simulink model "buck_hvoltage_discrete"  (R2014a)
settings: Solver=ode45  StartTime=0.0  StopTime=5*Tmax  RelTol=1e-3
values from neighbouring files (symbols this model uses):
  a00c = sys(1).Ac(1,1)    [parameters.m]
  a00d = sys(1).Ad(1,1)    [parameters.m]
  a00o = sys(1).Ao(1,1)    [parameters.m]
  a01c = sys(1).Ac(1,2)    [parameters.m]
  a01d = sys(1).Ad(1,2)    [parameters.m]
  a01o = sys(1).Ao(1,2)    [parameters.m]
  a10c = sys(1).Ac(2,1)    [parameters.m]
  a10d = sys(1).Ad(2,1)    [parameters.m]
  a10o = sys(1).Ao(2,1)    [parameters.m]
  a11c = sys(1).Ac(2,2)    [parameters.m]
  a11d = sys(1).Ad(2,2)    [parameters.m]
  a11o = sys(1).Ao(2,2)    [parameters.m]
  b0c = sys(1).Bc(1)    [parameters.m]
  b0d = sys(1).Bd(1)    [parameters.m]
  b0o = sys(1).Bo(1)    [parameters.m]
  b1c = sys(1).Bc(2)    [parameters.m]
  b1d = sys(1).Bd(2)    [parameters.m]
  b1o = sys(1).Bo(2)    [parameters.m]
  D = cr*Vref/(cr*Vref + Vs)    (= 0.489795918367)    [parameters.m]
  i0 = 4.5    [parameters.m]
  T = 4e-6    (= 4e-06)    [parameters.m]
  v0 = 48    [parameters.m]
  Vref = 15    [parameters.m]    (also in parameters_dcmicrogrid.m = [48 48]; parameters_dcmicrogrid_hynger.m = [48 48])
  Vtol = Vref / 200    (= 0.075)    [parameters.m]
libraries: simulink x1
settings Model: BufferReuse=off  Creator=Luan Nguyen  LastModifiedBy=tjohnson
settings DataIOCC: SignalLoggingSaveFormat=ModelDataLogs
settings OptimizationCC: OptimizeBlockIOStorage=off  BufferReuse=off  GlobalBufferReuse=off  ExpressionFolding=off  ExpressionDepthLimit=2147483647  LocalBlockOutputs=off
settings DebuggingCC: UnderspecifiedInitializationDetection=Classic  MaxConsecutiveZCsMsg=none  MultiTaskDSMMsg=warning  MultiTaskCondExecSysMsg=none  StateNameClashWarn=warning
settings RTWCC: IncludeERTFirstTime=on

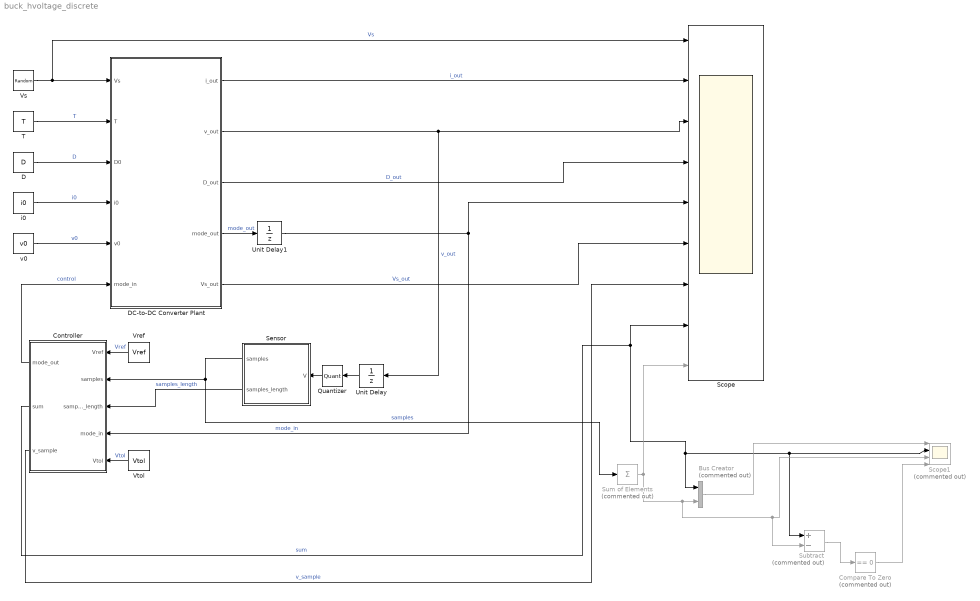
== system buck_hvoltage_discrete ==
  Bus Creator : BusCreator  Commented=on  Inputs=2
  Compare To Zero : simulink/Logic and Bit Operations/Compare To Zero  Commented=on  relop===  OutDataTypeStr=boolean
  Controller : Stateflow chart  TreatAsAtomicUnit=on
  D : Constant  Value=D
  DC-to-DC Converter Plant : Stateflow chart  TreatAsAtomicUnit=on
  Quantizer : Quantizer  QuantizationInterval=1
  Scope : Scope  NumInputPorts=9
      settings: TimeRange=0.00833333  YMin=95~-2.5e-12~46.1782~0.57684~1~95~46.55~744.8~-1  YMax=105~2.5e-12~51.039~0.63756~3~105~51.45~823.2000000000001~1  SaveName=dc2dc_ScopeData
  Scope1 : Scope  Commented=on  NumInputPorts=4
      settings: YMin=-5~-5~-5~-5  YMax=5~5~5~5
  Sensor : Stateflow chart  TreatAsAtomicUnit=on
  Subtract : Sum  Commented=on  Inputs=+-
  Sum of Elements : Sum  Commented=on  Inputs=+
  T : Constant  Value=T
  Unit Delay : UnitDelay  SampleTime=-1
  Unit Delay1 : UnitDelay  SampleTime=-1
  Vref : Constant  Value=Vref
  Vs : RandomNumber  Mean=100  Variance=15  SampleTime=T*100
  Vtol : Constant  Value=Vtol
  i0 : Constant  Value=i0
  v0 : Constant  Value=v0
  wires:
  DC-to-DC Converter Plant/1(i_out) -> Scope/2  "i_out"
  DC-to-DC Converter Plant/2(v_out) -> Unit Delay/1, Scope/3  "v_out"
  T/1 -> DC-to-DC Converter Plant/2(T)  "T"
  Vs/1 -> DC-to-DC Converter Plant/1(Vs), Scope/1  "Vs"
  i0/1 -> DC-to-DC Converter Plant/4(i0)  "i0"
  v0/1 -> DC-to-DC Converter Plant/5(v0)  "v0"
  D/1 -> DC-to-DC Converter Plant/3(D0)  "D"
  Vref/1 -> Controller/1(Vref)  "Vref"
  DC-to-DC Converter Plant/3(D_out) -> Scope/4  "D_out"
  DC-to-DC Converter Plant/4(mode_out) -> Unit Delay1/1  "mode_out"
  Vtol/1 -> Controller/5(Vtol)  "Vtol"
  DC-to-DC Converter Plant/5(Vs_out) -> Scope/6  "Vs_out"
  Controller/1(mode_out) -> DC-to-DC Converter Plant/6(mode_in)  "control"
  Unit Delay1/1 -> Controller/4(mode_in), Scope/5  "mode_in"
  Sensor/2(samples_length) -> Controller/3(samples_length)  "samples_length"
  Sensor/1(samples) -> Sum of Elements/1, Controller/2(samples)  "samples"
  Controller/3(v_sample) -> Scope/7  "v_sample"
  Controller/2(sum) -> Subtract/1, Scope1/2, Bus Creator/1, Scope/8  "sum"
  Unit Delay/1 -> Quantizer/1
  Quantizer/1 -> Sensor/1(V)
  Sum of Elements/1 -> Subtract/2, Scope1/3, Bus Creator/2, Scope/9
  Bus Creator/1 -> Scope1/1
  Subtract/1 -> Compare To Zero/1
  Compare To Zero/1 -> Scope1/4

== stateflow chart buck_hvoltage_discrete/DC-to-DC Converter Plant ==
  settings: updateMethod=CONTINUOUS
  state Discontinuous
    du:
    i_dot = a00d*i+a01d*v+b0d*Vs;
    v_dot = a10d*i+a11d*v+b1d*Vs;
    t_dot = 1;
    i_out =i;
    v_out = v;
    D_out=D;
    mode_out=3;
    Vs_out=Vs;
  state Charging
    du:
    i_dot = a00c*i+a01c*v+b0c*Vs;
    v_dot = a10c*i+a11c*v+b1c*Vs;
    t_dot = 1;
    i_out = i;
    v_out = v;
    D_out=D;
    mode_out=2;
    Vs_out=Vs;
  state Discharging
    du:
    i_dot = a00o*i+a01o*v+b0o*Vs;
    v_dot = a10o*i+a11o*v+b1o*Vs;
    t_dot = 1;
    i_out = i;
    v_out = v;
    D_out=D;
    mode_out=1;
    Vs_out=Vs;
  Discharging -> Discontinuous [order 1] : [i<=0]
  Discontinuous -> Charging : [mode_in==2]
      | //[i>=0.1]
      | //[t>=(1-D)*T]
      | {t=0;}
  Charging -> Discharging : [mode_in==1]
      | //&&t>=D*T
      | {t= 0;}
  Discharging -> Charging [order 2] : [mode_in==2]
      | //t>=(1-D)*T
      | {t= 0;}
  (default) -> Charging : {i = i0;
      | v = v0;
      | D=D0;}
  data: t local double; i_out output double; v_out output double; i local double; a00o local double; Vs input double =120; T input double; D0 input double; a01o local double; a10o local double; a11o local double; a00c local double; a01c local double; a10c local double; a11c local double; b0o local double; b1o local double; b0c local double; b1c local double; v local double; i0 input double; v0 input double; a01d local double; a10d local double; a11d local double; a00d local double; b0d local double; b1d local double; D local double; v1 local double; D_out output double; mode_out output double; Vs_out output double; mode_in input double =120
  data t settings: updateMethod=SF_CONTINUOUS_TIME_DATA
  data i settings: updateMethod=SF_CONTINUOUS_TIME_DATA
  data v settings: updateMethod=SF_CONTINUOUS_TIME_DATA
  data D settings: updateMethod=SF_CONTINUOUS_TIME_DATA
  data v1 settings: updateMethod=SF_CONTINUOUS_TIME_DATA

== stateflow chart buck_hvoltage_discrete/Sensor ==
  settings: updateMethod=DISCRETE  sampleTime=T
  state Sample
  state Hold
  (default) -> Sample : {samples_length=16;
      | index=0;}
  (junction 84) -> Sample : // reset circular buffer
      | {index=0;}
  Sample -> (junction 88)
  Hold -> (junction 85) [order 1] : [index<samples_length]
  (junction 88) -> Hold
  (junction 85) -> (junction 86) : {samples[index]=V;}
  Hold -> (junction 84) [order 2]
  (junction 86) -> Hold : {index++;}
  data: V input; samples output int32 size=16; samples_length output int32 size=1; index local int32

== stateflow chart buck_hvoltage_discrete/Controller ==
  settings: updateMethod=DISCRETE  sampleTime=T
  state Discharging
    entry: mode_out=1;
  state Hysteresis
    entry: mode_out = mode_in;
  state Charging
    entry: mode_out=2;
  (default) -> (junction 111) : // compute average of samples
  Hysteresis -> (junction 111)
  Discharging -> (junction 111)
  (junction 120) -> (junction 124) [order 1] : [index<samples_length]
  (junction 124) -> (junction 108) : {sum=sum+samples[index];}
  Charging -> (junction 111)
  (junction 111) -> (junction 120) : {index= 0;
      | sum=0;
      | v_sample=Vref;}
      | // last just for plotting
  (junction 108) -> (junction 120) : {index = index + 1;}
  (junction 120) -> (junction 117) [order 2] : {v_sample=sum/samples_length;}
  (junction 117) -> Hysteresis [order 3] : // default: stay same
  (junction 117) -> Charging [order 1] : [v_sample<=(Vref-Vtol)]
  (junction 117) -> Discharging [order 2] : [v_sample>=(Vref+Vtol)]
  data: Vref input; samples input; samples_length input; mode_in input; mode_out output; index local uint32 size=1; sum output int32 size=1; Vtol input; v_sample output double size=1
